simulink model "model_v4"  (R2023b)
settings: Solver=VariableStepAuto  StartTime=0.0  StopTime=10.0  RelTol=1e-3
(part 2 of 2)

== matlab function model_v4/MATLAB Function2 ==
  data: M input; y_m2_ddot output; m1 input; m2 input; m3 input; theta_m2 input; theta_m3 input; theta_M input; y_m2 input; y_M input; theta_m2_dot input; theta_m3_dot input; y_m2_dot input; y_M_dot input; y_M_ddot input; l1 input; l2 input; l3 input; r input; k1 input; k2 input; k3 input; k4 input; k5 input; c4 input; c5 input; Q3 input
function y_m2_ddot = y_m2(M, m1, m2, m3, theta_m2, theta_m3, theta_M, y_m2, y_M, theta_m2_dot, theta_m3_dot, y_m2_dot, y_M_dot, y_M_ddot, l1, l2, l3, r, k1, k2, k3, k4, k5, c4, c5, Q3)

g = 9.81;
y_m2_ddot = (M*g*sqrt((l3*sin(theta_m3) - y_M*tan(theta_M) + y_m2*tan(theta_M))^2 + (l1*theta_m2 + l3*cos(theta_m3) - y_M - y_m2)^2)*(l3*sin(theta_m3) - y_M*tan(theta_M) + y_m2*tan(theta_M))^2*cos(theta_M)*tan(theta_M) - M*g*sqrt((l3*sin(theta_m3) - y_M*tan(theta_M) + y_m2*tan(theta_M))^2 + (l1*theta_m2 + l3*cos(theta_m3) - y_M - y_m2)^2)*(l3*sin(theta_m3) - y_M*tan(theta_M) + y_m2*tan(theta_M))^2*tan(theta_M)^2 + M*g*sqrt((l3*sin(theta_m3) - y_M*tan(theta_M) + y_m2*tan(theta_M))^2 + (l1*theta_m2 + l3*cos(theta_m3) - y_M - y_m2)^2)*(l1*theta_m2 + l3*cos(theta_m3) - y_M - y_m2)^2*cos(theta_M)*tan(theta_M) - M*g*sqrt((l3*sin(theta_m3) - y_M*tan(theta_M) + y_m2*tan(theta_M))^2 + (l1*theta_m2 + l3*cos(theta_m3) - y_M - y_m2)^2)*(l1*theta_m2 + l3*cos(theta_m3) - y_M - y_m2)^2*tan(theta_M)^2 + Q3*sqrt((l3*sin(theta_m3) - y_M*tan(theta_M) + y_m2*tan(theta_M))^2 + (l1*theta_m2 + l3*cos(theta_m3) - y_M - y_m2)^2)*(l3*sin(theta_m3) - y_M*tan(theta_M) + y_m2*tan(theta_M))^2*tan(theta_M)^2 + Q3*sqrt((l3*sin(theta_m3) - y_M*tan(theta_M) + y_m2*tan(theta_M))^2 + (l1*theta_m2 + l3*cos(theta_m3) - y_M - y_m2)^2)*(l1*theta_m2 + l3*cos(theta_m3) - y_M - y_m2)^2*tan(theta_M)^2 + c4*l1^3*theta_m2^2*theta_m2_dot*sqrt((l3*sin(theta_m3) - y_M*tan(theta_M) + y_m2*tan(theta_M))^2 + (l1*theta_m2 + l3*cos(theta_m3) - y_M - y_m2)^2)*tan(theta_M)^2 - c4*l1^2*l3*theta_m2^2*theta_m3_dot*sqrt((l3*sin(theta_m3) - y_M*tan(theta_M) + y_m2*tan(theta_M))^2 + (l1*theta_m2 + l3*cos(theta_m3) - y_M - y_m2)^2)*sin(theta_m3)*tan(theta_M)^2 - c4*l1^2*l3*theta_m2*theta_m2_dot*sqrt((l3*sin(theta_m3) - y_M*tan(theta_M) + y_m2*tan(theta_M))^2 + (l1*theta_m2 + l3*cos(theta_m3) - y_M - y_m2)^2)*sin(theta_m3)*tan(theta_M)^3 + 2.0*c4*l1^2*l3*theta_m2*theta_m2_dot*sqrt((l3*sin(theta_m3) - y_M*tan(theta_M) + y_m2*tan(theta_M))^2 + (l1*theta_m2 + l3*cos(theta_m3) - y_M - y_m2)^2)*cos(theta_m3)*tan(theta_M)^2 - c4*l1^2*theta_m2^2*y_M_dot*sqrt((l3*sin(theta_m3) - y_M*tan(theta_M) + y_m2*tan(theta_M))^2 + (l1*theta_m2 + l3*cos(theta_m3) - y_M - y_m2)^2)*tan(theta_M)^2 - c4*l1^2*theta_m2^2*y_m2_dot*sqrt((l3*sin(theta_m3) - y_M*tan(theta_M) + y_m2*tan(theta_M))^2 + (l1*theta_m2 + l3*cos(theta_m3) - y_M - y_m2)^2)*tan(theta_M)^2 + c4*l1^2*theta_m2*theta_m2_dot*y_M*sqrt((l3*sin(theta_m3) - y_M*tan(theta_M) + y_m2*tan(theta_M))^2 + (l1*theta_m2 + l3*cos(theta_m3) - y_M - y_m2)^2)*tan(theta_M)^4 - 2.0*c4*l1^2*theta_m2*theta_m2_dot*y_M*sqrt((l3*sin(theta_m3) - y_M*tan(theta_M) + y_m2*tan(theta_M))^2 + (l1*theta_m2 + l3*cos(theta_m3) - y_M - y_m2)^2)*tan(theta_M)^2 - c4*l1^2*theta_m2*theta_m2_dot*y_m2*sqrt((l3*sin(theta_m3) - y_M*tan(theta_M) + y_m2*tan(theta_M))^2 + (l1*theta_m2 + l3*cos(theta_m3) - y_M - y_m2)^2)*tan(theta_M)^4 - 2.0*c4*l1^2*theta_m2*theta_m2_dot*y_m2*sqrt((l3*sin(theta_m3) - y_M*tan(theta_M) + y_m2*tan(theta_M))^2 + (l1*theta_m2 + l3*cos(theta_m3) - y_M - y_m2)^2)*tan(theta_M)^2 + c4*l1*l3^2*theta_m2*theta_m3_dot*sqrt((l3*sin(theta_m3) - y_M*tan(theta_M) + y_m2*tan(theta_M))^2 + (l1*theta_m2 + l3*cos(theta_m3) - y_M - y_m2)^2)*sin(theta_m3)^2*tan(theta_M)^3 - c4*l1*l3^2*theta_m2*theta_m3_dot*sqrt((l3*sin(theta_m3) - y_M*tan(theta_M) + y_m2*tan(theta_M))^2 + (l1*theta_m2 + l3*cos(theta_m3) - y_M - y_m2)^2)*sin(theta_m3)*cos(theta_m3)*tan(theta_M)^2 - c4*l1*l3^2*theta_m2_dot*sqrt((l3*sin(theta_m3) - y_M*tan(theta_M) + y_m2*tan(theta_M))^2 + (l1*theta_m2 + l3*cos(theta_m3) - y_M - y_m2)^2)*sin(theta_m3)*cos(theta_m3)*tan(theta_M)^3 + c4*l1*l3^2*theta_m2_dot*sqrt((l3*sin(theta_m3) - y_M*tan(theta_M) + y_m2*tan(theta_M))^2 + (l1*theta_m2 + l3*cos(theta_m3) - y_M - y_m2)^2)*cos(theta_m3)^2*tan(theta_M)^2 - c4*l1*l3*theta_m2*theta_m3_dot*y_M*sqrt((l3*sin(theta_m3) - y_M*tan(theta_M) + y_m2*tan(theta_M))^2 + (l1*theta_m2 + l3*cos(theta_m3) - y_M - y_m2)^2)*sin(theta_m3)*tan(theta_M)^4 + 2.0*c4*l1*l3*theta_m2*theta_m3_dot*y_M*sqrt((l3*sin(theta_m3) - y_M*tan(theta_M) + y_m2*tan(theta_M))^2 + (l1*theta_m2 + l3*cos(theta_m3) - y_M - y_m2)^2)*sin(theta_m3)*tan(theta_M)^2 - c4*l1*l3*theta_m2*theta_m3_dot*y_M*sqrt((l3*sin(theta_m3) - y_M*tan(theta_M) + y_m2*tan(theta_M))^2 + (l1*theta_m2 + l3*cos(theta_m3) - y_M - y_m2)^2)*cos(theta_m3)*tan(theta_M)^3 + c4*l1*l3*theta_m2*theta_m3_dot*y_m2*sqrt((l3*sin(theta_m3) - y_M*tan(theta_M) + y_m2*tan(theta_M))^2 + (l1*theta_m2 + l3*cos(theta_m3) - y_M - y_m2)^2)*sin(theta_m3)*tan(theta_M)^4 + 2.0*c4*l1*l3*theta_m2*theta_m3_dot*y_m2*sqrt((l3*sin(theta_m3) - y_M*tan(theta_M) + y_m2*tan(theta_M))^2 + (l1*theta_m2 + l3*cos(theta_m3) - y_M - y_m2)^2)*sin(theta_m3)*tan(theta_M)^2 + c4*l1*l3*theta_m2*theta_m3_dot*y_m2*sqrt((l3*sin(theta_m3) - y_M*tan(theta_M) + y_m2*tan(theta_M))^2 + (l1*theta_m2 + l3*cos(theta_m3) - y_M - y_m2)^2)*cos(theta_m3)*tan(theta_M)^3 - 2.0*c4*l1*l3*theta_m2*y_M_dot*sqrt((l3*sin(theta_m3) - y_M*tan(theta_M) + y_m2*tan(theta_M))^2 + (l1*theta_m2 + l3*cos(theta_m3) - y_M - y_m2)^2)*cos(theta_m3)*tan(theta_M)^2 + 2.0*c4*l1*l3*theta_m2*y_m2_dot*sqrt((l3*sin(theta_m3) - y_M*tan(theta_M) + y_m2*tan(theta_M))^2 + (l1*theta_m2 + l3*cos(theta_m3) - y_M - y_m2)^2)*sin(theta_m3)*tan(theta_M)^3 - 2.0*c4*l1*l3*theta_m2*y_m2_dot*sqrt((l3*sin(theta_m3) - y_M*tan(theta_M) + y_m2*tan(theta_M))^2 + (l1*theta_m2 + l3*cos(theta_m3) - y_M - y_m2)^2)*cos(theta_m3)*tan(theta_M)^2 + c4*l1*l3*theta_m2_dot*y_M*sqrt((l3*sin(theta_m3) - y_M*tan(theta_M) + y_m2*tan(theta_M))^2 + (l1*theta_m2 + l3*cos(theta_m3) - y_M - y_m2)^2)*sin(theta_m3)*tan(theta_M)^3 + c4*l1*l3*theta_m2_dot*y_M*sqrt((l3*sin(theta_m3) - y_M*tan(theta_M) + y_m2*tan(theta_M))^2 + (l1*theta_m2 + l3*cos(theta_m3) - y_M - y_m2)^2)*cos(theta_m3)*tan(theta_M)^4 - 2.0*c4*l1*l3*theta_m2_dot*y_M*sqrt((l3*sin(theta_m3) - y_M*tan(theta_M) + y_m2*tan(theta_M))^2 + (l1*theta_m2 + l3*cos(theta_m3) - y_M - y_m2)^2)*cos(theta_m3)*tan(theta_M)^2 + c4*l1*l3*theta_m2_dot*y_m2*sqrt((l3*sin(theta_m3) - y_M*tan(theta_M) + y_m2*tan(theta_M))^2 + (l1*theta_m2 + l3*cos(theta_m3) - y_M - y_m2)^2)*sin(theta_m3)*tan(theta_M)^3 - c4*l1*l3*theta_m2_dot*y_m2*sqrt((l3*sin(theta_m3) - y_M*tan(theta_M) + y_m2*tan(theta_M))^2 + (l1*theta_m2 + l3*cos(theta_m3) - y_M - y_m2)^2)*cos(theta_m3)*tan(theta_M)^4 - 2.0*c4*l1*l3*theta_m2_dot*y_m2*sqrt((l3*sin(theta_m3) - y_M*tan(theta_M) + y_m2*tan(theta_M))^2 + (l1*theta_m2 + l3*cos(theta_m3) - y_M - y_m2)^2)*cos(theta_m3)*tan(theta_M)^2 + 2.0*c4*l1*theta_m2*y_M*y_M_dot*sqrt((l3*sin(theta_m3) - y_M*tan(theta_M) + y_m2*tan(theta_M))^2 + (l1*theta_m2 + l3*cos(theta_m3) - y_M - y_m2)^2)*tan(theta_M)^2 - 2.0*c4*l1*theta_m2*y_M*y_m2_dot*sqrt((l3*sin(theta_m3) - y_M*tan(theta_M) + y_m2*tan(theta_M))^2 + (l1*theta_m2 + l3*cos(theta_m3) - y_M - y_m2)^2)*tan(theta_M)^4 + 2.0*c4*l1*theta_m2*y_M*y_m2_dot*sqrt((l3*sin(theta_m3) - y_M*tan(theta_M) + y_m2*tan(theta_M))^2 + (l1*theta_m2 + l3*cos(theta_m3) - y_M - y_m2)^2)*tan(theta_M)^2 + 2.0*c4*l1*theta_m2*y_M_dot*y_m2*sqrt((l3*sin(theta_m3) - y_M*tan(theta_M) + y_m2*tan(theta_M))^2 + (l1*theta_m2 + l3*cos(theta_m3) - y_M - y_m2)^2)*tan(theta_M)^2 + 2.0*c4*l1*theta_m2*y_m2*y_m2_dot*sqrt((l3*sin(theta_m3) - y_M*tan(theta_M) + y_m2*tan(theta_M))^2 + (l1*theta_m2 + l3*cos(theta_m3) - y_M - y_m2)^2)*tan(theta_M)^4 + 2.0*c4*l1*theta_m2*y_m2*y_m2_dot*sqrt((l3*sin(theta_m3) - y_M*tan(theta_M) + y_m2*tan(theta_M))^2 + (l1*theta_m2 + l3*cos(theta_m3) - y_M - y_m2)^2)*tan(theta_M)^2 - c4*l1*theta_m2_dot*y_M^2*sqrt((l3*sin(theta_m3) - y_M*tan(theta_M) + y_m2*tan(theta_M))^2 + (l1*theta_m2 + l3*cos(theta_m3) - y_M - y_m2)^2)*tan(theta_M)^4 + c4*l1*theta_m2_dot*y_M^2*sqrt((l3*sin(theta_m3) - y_M*tan(theta_M) + y_m2*tan(theta_M))^2 + (l1*theta_m2 + l3*cos(theta_m3) - y_M - y_m2)^2)*tan(theta_M)^2 + 2.0*c4*l1*theta_m2_dot*y_M*y_m2*sqrt((l3*sin(theta_m3) - y_M*tan(theta_M) + y_m2*tan(theta_M))^2 + (l1*theta_m2 + l3*cos(theta_m3) - y_M - y_m2)^2)*tan(theta_M)^2 + c4*l1*theta_m2_dot*y_m2^2*sqrt((l3*sin(theta_m3) - y_M*tan(theta_M) + y_m2*tan(theta_M))^2 + (l1*theta_m2 + l3*cos(theta_m3) - y_M - y_m2)^2)*tan(theta_M)^4 + c4*l1*theta_m2_dot*y_m2^2*sqrt((l3*sin(theta_m3) - y_M*tan(theta_M) + y_m2*tan(theta_M))^2 + (l1*theta_m2 + l3*cos(theta_m3) - y_M - y_m2)^2)*tan(theta_M)^2 - c4*l3^2*theta_m3_dot*y_M*sqrt((l3*sin(theta_m3) - y_M*tan(theta_M) + y_m2*tan(theta_M))^2 + (l1*theta_m2 + l3*cos(theta_m3) - y_M - y_m2)^2)*sin(theta_m3)^2*tan(theta_M)^3 + c4*l3^2*theta_m3_dot*y_M*sqrt((l3*sin(theta_m3) - y_M*tan(theta_M) + y_m2*tan(theta_M))^2 + (l1*theta_m2 + l3*cos(theta_m3) - y_M - y_m2)^2)*sin(theta_m3)*cos(theta_m3)*tan(theta_M)^4 + c4*l3^2*theta_m3_dot*y_M*sqrt((l3*sin(theta_m3) - y_M*tan(theta_M) + y_m2*tan(theta_M))^2 + (l1*theta_m2 + l3*cos(theta_m3) - y_M - y_m2)^2)*sin(theta_m3)*cos(theta_m3)*tan(theta_M)^2 - c4*l3^2*theta_m3_dot*y_M*sqrt((l3*sin(theta_m3) - y_M*tan(theta_M) + y_m2*tan(theta_M))^2 + (l1*theta_m2 + l3*cos(theta_m3) - y_M - y_m2)^2)*cos(theta_m3)^2*tan(theta_M)^3 - c4*l3^2*theta_m3_dot*y_m2*sqrt((l3*sin(theta_m3) - y_M*tan(theta_M) + y_m2*tan(theta_M))^2 + (l1*theta_m2 + l3*cos(theta_m3) - y_M - y_m2)^2)*sin(theta_m3)^2*tan(theta_M)^3 - c4*l3^2*theta_m3_dot*y_m2*sqrt((l3*sin(theta_m3) - y_M*tan(theta_M) + y_m2*tan(theta_M))^2 + (l1*theta_m2 + l3*cos(theta_m3) - y_M - y_m2)^2)*sin(theta_m3)*cos(theta_m3)*tan(theta_M)^4 + c4*l3^2*theta_m3_dot*y_m2*sqrt((l3*sin(theta_m3) - y_M*tan(theta_M) + y_m2*tan(theta_M))^2 + (l1*theta_m2 + l3*cos(theta_m3) - y_M - y_m2)^2)*sin(theta_m3)*cos(theta_m3)*tan(theta_M)^2 + c4*l3^2*theta_m3_dot*y_m2*sqrt((l3*sin(theta_m3) - y_M*tan(theta_M) + y_m2*tan(theta_M))^2 + (l1*theta_m2 + l3*cos(theta_m3) - y_M - y_m2)^2)*cos(theta_m3)^2*tan(theta_M)^3 + c4*l3^2*y_M_dot*sqrt((l3*sin(theta_m3) - y_M*tan(theta_M) + y_m2*tan(theta_M))^2 + (l1*theta_m2 + l3*cos(theta_m3) - y_M - y_m2)^2)*sin(theta_m3)^2*tan(theta_M)^4 - c4*l3^2*y_M_dot*sqrt((l3*sin(theta_m3) - y_M*tan(theta_M) + y_m2*tan(theta_M))^2 + (l1*theta_m2 + l3*cos(theta_m3) - y_M - y_m2)^2)*cos(theta_m3)^2*tan(theta_M)^2 - c4*l3^2*y_m2_dot*sqrt((l3*sin(theta_m3) - y_M*tan(theta_M) + y_m2*tan(theta_M))^2 + (l1*theta_m2 + l3*cos(theta_m3) - y_M - y_m2)^2)*sin(theta_m3)^2*tan(theta_M)^4 + 2.0*c4*l3^2*y_m2_dot*sqrt((l3*sin(theta_m3) - y_M*tan(theta_M) + y_m2*tan(theta_M))^2 + (l1*theta_m2 + l3*cos(theta_m3) - y_M - y_m2)^2)*sin(theta_m3)*cos(theta_m3)*tan(theta_M)^3 - c4*l3^2*y_m2_dot*sqrt((l3*sin(theta_m3) - y_M*tan(theta_M) + y_m2*tan(theta_M))^2 + (l1*theta_m2 + l3*cos(theta_m3) - y_M - y_m2)^2)*cos(theta_m3)^2*tan(theta_M)^2 + c4*l3*theta_m3_dot*y_M^2*sqrt((l3*sin(theta_m3) - y_M*tan(theta_M) + y_m2*tan(theta_M))^2 + (l1*theta_m2 + l3*cos(theta_m3) - y_M - y_m2)^2)*sin(theta_m3)*tan(theta_M)^4 - c4*l3*theta_m3_dot*y_M^2*sqrt((l3*sin(theta_m3) - y_M*tan(theta_M) + y_m2*tan(theta_M))^2 + (l1*theta_m2 + l3*cos(theta_m3) - y_M - y_m2)^2)*sin(theta_m3)*tan(theta_M)^2 - c4*l3*theta_m3_dot*y_M^2*sqrt((l3*sin(theta_m3) - y_M*tan(theta_M) + y_m2*tan(theta_M))^2 + (l1*theta_m2 + l3*cos(theta_m3) - y_M - y_m2)^2)*cos(theta_m3)*tan(theta_M)^5 + c4*l3*theta_m3_dot*y_M^2*sqrt((l3*sin(theta_m3) - y_M*tan(theta_M) + y_m2*tan(theta_M))^2 + (l1*theta_m2 + l3*cos(theta_m3) - y_M - y_m2)^2)*cos(theta_m3)*tan(theta_M)^3 - 2.0*c4*l3*theta_m3_dot*y_M*y_m2*sqrt((l3*sin(theta_m3) - y_M*tan(theta_M) + y_m2*tan(theta_M))^2 + (l1*theta_m2 + l3*cos(theta_m3) - y_M - y_m2)^2)*sin(theta_m3)*tan(theta_M)^2 + 2.0*c4*l3*theta_m3_dot*y_M*y_m2*sqrt((l3*sin(theta_m3) - y_M*tan(theta_M) + y_m2*tan(theta_M))^2 + (l1*theta_m2 + l3*cos(theta_m3) - y_M - y_m2)^2)*cos(theta_m3)*tan(theta_M)^5 - c4*l3*theta_m3_dot*y_m2^2*sqrt((l3*sin(theta_m3) - y_M*tan(theta_M) + y_m2*tan(theta_M))^2 + (l1*theta_m2 + l3*cos(theta_m3) - y_M - y_m2)^2)*sin(theta_m3)*tan(theta_M)^4 - c4*l3*theta_m3_dot*y_m2^2*sqrt((l3*sin(theta_m3) - y_M*tan(theta_M) + y_m2*tan(theta_M))^2 + (l1*theta_m2 + l3*cos(theta_m3) - y_M - y_m2)^2)*sin(theta_m3)*tan(theta_M)^2 - c4*l3*theta_m3_dot*y_m2^2*sqrt((l3*sin(theta_m3) - y_M*tan(theta_M) + y_m2*tan(theta_M))^2 + (l1*theta_m2 + l3*cos(theta_m3) - y_M - y_m2)^2)*cos(theta_m3)*tan(theta_M)^5 - c4*l3*theta_m3_dot*y_m2^2*sqrt((l3*sin(theta_m3) - y_M*tan(theta_M) + y_m2*tan(theta_M))^2 + (l1*theta_m2 + l3*cos(theta_m3) - y_M - y_m2)^2)*cos(theta_m3)*tan(theta_M)^3 - 2.0*c4*l3*y_M*y_M_dot*sqrt((l3*sin(theta_m3) - y_M*tan(theta_M) + y_m2*tan(theta_M))^2 + (l1*theta_m2 + l3*cos(theta_m3) - y_M - y_m2)^2)*sin(theta_m3)*tan(theta_M)^5 + 2.0*c4*l3*y_M*y_M_dot*sqrt((l3*sin(theta_m3) - y_M*tan(theta_M) + y_m2*tan(theta_M))^2 + (l1*theta_m2 + l3*cos(theta_m3) - y_M - y_m2)^2)*cos(theta_m3)*tan(theta_M)^2 + 2.0*c4*l3*y_M*y_m2_dot*sqrt((l3*sin(theta_m3) - y_M*tan(theta_M) + y_m2*tan(theta_M))^2 + (l1*theta_m2 + l3*cos(theta_m3) - y_M - y_m2)^2)*sin(theta_m3)*tan(theta_M)^5 - 2.0*c4*l3*y_M*y_m2_dot*sqrt((l3*sin(theta_m3) - y_M*tan(theta_M) + y_m2*tan(theta_M))^2 + (l1*theta_m2 + l3*cos(theta_m3) - y_M - y_m2)^2)*sin(theta_m3)*tan(theta_M)^3 - 2.0*c4*l3*y_M*y_m2_dot*sqrt((l3*sin(theta_m3) - y_M*tan(theta_M) + y_m2*tan(theta_M))^2 + (l1*theta_m2 + l3*cos(theta_m3) - y_M - y_m2)^2)*cos(theta_m3)*tan(theta_M)^4 + 2.0*c4*l3*y_M*y_m2_dot*sqrt((l3*sin(theta_m3) - y_M*tan(theta_M) + y_m2*tan(theta_M))^2 + (l1*theta_m2 + l3*cos(theta_m3) - y_M - y_m2)^2)*cos(theta_m3)*tan(theta_M)^2 + 2.0*c4*l3*y_M_dot*y_m2*sqrt((l3*sin(theta_m3) - y_M*tan(theta_M) + y_m2*tan(theta_M))^2 + (l1*theta_m2 + l3*cos(theta_m3) - y_M - y_m2)^2)*sin(theta_m3)*tan(theta_M)^5 + 2.0*c4*l3*y_M_dot*y_m2*sqrt((l3*sin(theta_m3) - y_M*tan(theta_M) + y_m2*tan(theta_M))^2 + (l1*theta_m2 + l3*cos(theta_m3) - y_M - y_m2)^2)*cos(theta_m3)*tan(theta_M)^2 - 2.0*c4*l3*y_m2*y_m2_dot*sqrt((l3*sin(theta_m3) - y_M*tan(theta_M) + y_m2*tan(theta_M))^2 + (l1*theta_m2 + l3*cos(theta_m3) - y_M - y_m2)^2)*sin(theta_m3)*tan(theta_M)^5 - 2.0*c4*l3*y_m2*y_m2_dot*sqrt((l3*sin(theta_m3) - y_M*tan(theta_M) + y_m2*tan(theta_M))^2 + (l1*theta_m2 + l3*cos(theta_m3) - y_M - y_m2)^2)*sin(theta_m3)*tan(theta_M)^3 + 2.0*c4*l3*y_m2*y_m2_dot*sqrt((l3*sin(theta_m3) - y_M*tan(theta_M) + y_m2*tan(theta_M))^2 + (l1*theta_m2 + l3*cos(theta_m3) - y_M - y_m2)^2)*cos(theta_m3)*tan(theta_M)^4 + 2.0*c4*l3*y_m2*y_m2_dot*sqrt((l3*sin(theta_m3) - y_M*tan(theta_M) + y_m2*tan(theta_M))^2 + (l1*theta_m2 + l3*cos(theta_m3) - y_M - y_m2)^2)*cos(theta_m3)*tan(theta_M)^2 + c4*y_M^2*y_M_dot*sqrt((l3*sin(theta_m3) - y_M*tan(theta_M) + y_m2*tan(theta_M))^2 + (l1*theta_m2 + l3*cos(theta_m3) - y_M - y_m2)^2)*tan(theta_M)^6 - c4*y_M^2*y_M_dot*sqrt((l3*sin(theta_m3) - y_M*tan(theta_M) + y_m2*tan(theta_M))^2 + (l1*theta_m2 + l3*cos(theta_m3) - y_M - y_m2)^2)*tan(theta_M)^2 - c4*y_M^2*y_m2_dot*sqrt((l3*sin(theta_m3) - y_M*tan(theta_M) + y_m2*tan(theta_M))^2 + (l1*theta_m2 + l3*cos(theta_m3) - y_M - y_m2)^2)*tan(theta_M)^6 + 2.0*c4*y_M^2*y_m2_dot*sqrt((l3*sin(theta_m3) - y_M*tan(theta_M) + y_m2*tan(theta_M))^2 + (l1*theta_m2 + l3*cos(theta_m3) - y_M - y_m2)^2)*tan(theta_M)^4 - c4*y_M^2*y_m2_dot*sqrt((l3*sin(theta_m3) - y_M*tan(theta_M) + y_m2*tan(theta_M))^2 + (l1*theta_m2 + l3*cos(theta_m3) - y_M - y_m2)^2)*tan(theta_M)^2 - 2.0*c4*y_M*y_M_dot*y_m2*sqrt((l3*sin(theta_m3) - y_M*tan(theta_M) + y_m2*tan(theta_M))^2 + (l1*theta_m2 + l3*cos(theta_m3) - y_M - y_m2)^2)*tan(theta_M)^6 - 2.0*c4*y_M*y_M_dot*y_m2*sqrt((l3*sin(theta_m3) - y_M*tan(theta_M) + y_m2*tan(theta_M))^2 + (l1*theta_m2 + l3*cos(theta_m3) - y_M - y_m2)^2)*tan(theta_M)^2 + 2.0*c4*y_M*y_m2*y_m2_dot*sqrt((l3*sin(theta_m3) - y_M*tan(theta_M) + y_m2*tan(theta_M))^2 + (l1*theta_m2 + l3*cos(theta_m3) - y_M - y_m2)^2)*tan(theta_M)^6 - 2.0*c4*y_M*y_m2*y_m2_dot*sqrt((l3*sin(theta_m3) - y_M*tan(theta_M) + y_m2*tan(theta_M))^2 + (l1*theta_m2 + l3*cos(theta_m3) - y_M - y_m2)^2)*tan(theta_M)^2 + c4*y_M_dot*y_m2^2*sqrt((l3*sin(theta_m3) - y_M*tan(theta_M) + y_m2*tan(theta_M))^2 + (l1*theta_m2 + l3*cos(theta_m3) - y_M - y_m2)^2)*tan(theta_M)^6 - c4*y_M_dot*y_m2^2*sqrt((l3*sin(theta_m3) - y_M*tan(theta_M) + y_m2*tan(theta_M))^2 + (l1*theta_m2 + l3*cos(theta_m3) - y_M - y_m2)^2)*tan(theta_M)^2 - c4*y_m2^2*y_m2_dot*sqrt((l3*sin(theta_m3) - y_M*tan(theta_M) + y_m2*tan(theta_M))^2 + (l1*theta_m2 + l3*cos(theta_m3) - y_M - y_m2)^2)*tan(theta_M)^6 - 2.0*c4*y_m2^2*y_m2_dot*sqrt((l3*sin(theta_m3) - y_M*tan(theta_M) + y_m2*tan(theta_M))^2 + (l1*theta_m2 + l3*cos(theta_m3) - y_M - y_m2)^2)*tan(theta_M)^4 - c4*y_m2^2*y_m2_dot*sqrt((l3*sin(theta_m3) - y_M*tan(theta_M) + y_m2*tan(theta_M))^2 + (l1*theta_m2 + l3*cos(theta_m3) - y_M - y_m2)^2)*tan(theta_M)^2 + c5*y_M_dot*sqrt((l3*sin(theta_m3) - y_M*tan(theta_M) + y_m2*tan(theta_M))^2 + (l1*theta_m2 + l3*cos(theta_m3) - y_M - y_m2)^2)*(l3*sin(theta_m3) - y_M*tan(theta_M) + y_m2*tan(theta_M))^2 + c5*y_M_dot*sqrt((l3*sin(theta_m3) - y_M*tan(theta_M) + y_m2*tan(theta_M))^2 + (l1*theta_m2 + l3*cos(theta_m3) - y_M - y_m2)^2)*(l1*theta_m2 + l3*cos(theta_m3) - y_M - y_m2)^2 - c5*y_m2_dot*sqrt((l3*sin(theta_m3) - y_M*tan(theta_M) + y_m2*tan(theta_M))^2 + (l1*theta_m2 + l3*cos(theta_m3) - y_M - y_m2)^2)*(l3*sin(theta_m3) - y_M*tan(theta_M) + y_m2*tan(theta_M))^2 - c5*y_m2_dot*sqrt((l3*sin(theta_m3) - y_M*tan(theta_M) + y_m2*tan(theta_M))^2 + (l1*theta_m2 + l3*cos(theta_m3) - y_M - y_m2)^2)*(l1*theta_m2 + l3*cos(theta_m3) - y_M - y_m2)^2 - g*m1*sqrt((l3*sin(theta_m3) - y_M*tan(theta_M) + y_m2*tan(theta_M))^2 + (l1*theta_m2 + l3*cos(theta_m3) - y_M - y_m2)^2)*(l3*sin(theta_m3) - y_M*tan(theta_M) + y_m2*tan(theta_M))^2*tan(theta_M)^2 - g*m1*sqrt((l3*sin(theta_m3) - y_M*tan(theta_M) + y_m2*tan(theta_M))^2 + (l1*theta_m2 + l3*cos(theta_m3) - y_M - y_m2)^2)*(l1*theta_m2 + l3*cos(theta_m3) - y_M - y_m2)^2*tan(theta_M)^2 - g*m2*sqrt((l3*sin(theta_m3) - y_M*tan(theta_M) + y_m2*tan(theta_M))^2 + (l1*theta_m2 + l3*cos(theta_m3) - y_M - y_m2)^2)*(l3*sin(theta_m3) - y_M*tan(theta_M) + y_m2*tan(theta_M))^2*tan(theta_M)^2 - g*m2*sqrt((l3*sin(theta_m3) - y_M*tan(theta_M) + y_m2*tan(theta_M))^2 + (l1*theta_m2 + l3*cos(theta_m3) - y_M - y_m2)^2)*(l1*theta_m2 + l3*cos(theta_m3) - y_M - y_m2)^2*tan(theta_M)^2 - g*m3*sqrt((l3*sin(theta_m3) - y_M*tan(theta_M) + y_m2*tan(theta_M))^2 + (l1*theta_m2 + l3*cos(theta_m3) - y_M - y_m2)^2)*(l3*sin(theta_m3) - y_M*tan(theta_M) + y_m2*tan(theta_M))^2*tan(theta_M)^2 - g*m3*sqrt((l3*sin(theta_m3) - y_M*tan(theta_M) + y_m2*tan(theta_M))^2 + (l1*theta_m2 + l3*cos(theta_m3) - y_M - y_m2)^2)*(l1*theta_m2 + l3*cos(theta_m3) - y_M - y_m2)^2*tan(theta_M)^2 - k1*l1*sqrt((l3*sin(theta_m3) - y_M*tan(theta_M) + y_m2*tan(theta_M))^2 + (l1*theta_m2 + l3*cos(theta_m3) - y_M - y_m2)^2)*(l3*sin(theta_m3) - y_M*tan(theta_M) + y_m2*tan(theta_M))^2*sin(theta_m2)*tan(theta_M)^2 - k1*l1*sqrt((l3*sin(theta_m3) - y_M*tan(theta_M) + y_m2*tan(theta_M))^2 + (l1*theta_m2 + l3*cos(theta_m3) - y_M - y_m2)^2)*(l1*theta_m2 + l3*cos(theta_m3) - y_M - y_m2)^2*sin(theta_m2)*tan(theta_M)^2 - k1*y_m2*sqrt((l3*sin(theta_m3) - y_M*tan(theta_M) + y_m2*tan(theta_M))^2 + (l1*theta_m2 + l3*cos(theta_m3) - y_M - y_m2)^2)*(l3*sin(theta_m3) - y_M*tan(theta_M) + y_m2*tan(theta_M))^2*tan(theta_M)^2 - k1*y_m2*sqrt((l3*sin(theta_m3) - y_M*tan(theta_M) + y_m2*tan(theta_M))^2 + (l1*theta_m2 + l3*cos(theta_m3) - y_M - y_m2)^2)*(l1*theta_m2 + l3*cos(theta_m3) - y_M - y_m2)^2*tan(theta_M)^2 - k2*y_m2*sqrt((l3*sin(theta_m3) - y_M*tan(theta_M) + y_m2*tan(theta_M))^2 + (l1*theta_m2 + l3*cos(theta_m3) - y_M - y_m2)^2)*(l3*sin(theta_m3) - y_M*tan(theta_M) + y_m2*tan(theta_M))^2*tan(theta_M)^2 - k2*y_m2*sqrt((l3*sin(theta_m3) - y_M*tan(theta_M) + y_m2*tan(theta_M))^2 + (l1*theta_m2 + l3*cos(theta_m3) - y_M - y_m2)^2)*(l1*theta_m2 + l3*cos(theta_m3) - y_M - y_m2)^2*tan(theta_M)^2 + k3*l1*sqrt((l3*sin(theta_m3) - y_M*tan(theta_M) + y_m2*tan(theta_M))^2 + (l1*theta_m2 + l3*cos(theta_m3) - y_M - y_m2)^2)*(l3*sin(theta_m3) - y_M*tan(theta_M) + y_m2*tan(theta_M))^2*sin(theta_m2)*tan(theta_M)^2 + k3*l1*sqrt((l3*sin(theta_m3) - y_M*tan(theta_M) + y_m2*tan(theta_M))^2 + (l1*theta_m2 + l3*cos(theta_m3) - y_M - y_m2)^2)*(l1*theta_m2 + l3*cos(theta_m3) - y_M - y_m2)^2*sin(theta_m2)*tan(theta_M)^2 - k3*y_m2*sqrt((l3*sin(theta_m3) - y_M*tan(theta_M) + y_m2*tan(theta_M))^2 + (l1*theta_m2 + l3*cos(theta_m3) - y_M - y_m2)^2)*(l3*sin(theta_m3) - y_M*tan(theta_M) + y_m2*tan(theta_M))^2*tan(theta_M)^2 - k3*y_m2*sqrt((l3*sin(theta_m3) - y_M*tan(theta_M) + y_m2*tan(theta_M))^2 + (l1*theta_m2 + l3*cos(theta_m3) - y_M - y_m2)^2)*(l1*theta_m2 + l3*cos(theta_m3) - y_M - y_m2)^2*tan(theta_M)^2 - k4*l1*l3*theta_m2*(l3*sin(theta_m3) - y_M*tan(theta_M) + y_m2*tan(theta_M))^2*tan(theta_M)^2 - k4*l1*l3*theta_m2*(l1*theta_m2 + l3*cos(theta_m3) - y_M - y_m2)^2*tan(theta_M)^2 + k4*l1*theta_m2*sqrt((l3*sin(theta_m3) - y_M*tan(theta_M) + y_m2*tan(theta_M))^2 + (l1*theta_m2 + l3*cos(theta_m3) - y_M - y_m2)^2)*(l3*sin(theta_m3) - y_M*tan(theta_M) + y_m2*tan(theta_M))^2*tan(theta_M)^2 + k4*l1*theta_m2*sqrt((l3*sin(theta_m3) - y_M*tan(theta_M) + y_m2*tan(theta_M))^2 + (l1*theta_m2 + l3*cos(theta_m3) - y_M - y_m2)^2)*(l1*theta_m2 + l3*cos(theta_m3) - y_M - y_m2)^2*tan(theta_M)^2 + k4*l3^2*(l3*sin(theta_m3) - y_M*tan(theta_M) + y_m2*tan(theta_M))^2*sin(theta_m3)*tan(theta_M)^3 - k4*l3^2*(l3*sin(theta_m3) - y_M*tan(theta_M) + y_m2*tan(theta_M))^2*cos(theta_m3)*tan(theta_M)^2 + k4*l3^2*(l1*theta_m2 + l3*cos(theta_m3) - y_M - y_m2)^2*sin(theta_m3)*tan(theta_M)^3 - k4*l3^2*(l1*theta_m2 + l3*cos(theta_m3) - y_M - y_m2)^2*cos(theta_m3)*tan(theta_M)^2 - k4*l3*y_M*(l3*sin(theta_m3) - y_M*tan(theta_M) + y_m2*tan(theta_M))^2*tan(theta_M)^4 + k4*l3*y_M*(l3*sin(theta_m3) - y_M*tan(theta_M) + y_m2*tan(theta_M))^2*tan(theta_M)^2 - k4*l3*y_M*(l1*theta_m2 + l3*cos(theta_m3) - y_M - y_m2)^2*tan(theta_M)^4 + k4*l3*y_M*(l1*theta_m2 + l3*cos(theta_m3) - y_M - y_m2)^2*tan(theta_M)^2 + k4*l3*y_m2*(l3*sin(theta_m3) - y_M*tan(theta_M) + y_m2*tan(theta_M))^2*tan(theta_M)^4 + k4*l3*y_m2*(l3*sin(theta_m3) - y_M*tan(theta_M) + y_m2*tan(theta_M))^2*tan(theta_M)^2 + k4*l3*y_m2*(l1*theta_m2 + l3*cos(theta_m3) - y_M - y_m2)^2*tan(theta_M)^4 + k4*l3*y_m2*(l1*theta_m2 + l3*cos(theta_m3) - y_M - y_m2)^2*tan(theta_M)^2 - k4*l3*sqrt((l3*sin(theta_m3) - y_M*tan(theta_M) + y_m2*tan(theta_M))^2 + (l1*theta_m2 + l3*cos(theta_m3) - y_M - y_m2)^2)*(l3*sin(theta_m3) - y_M*tan(theta_M) + y_m2*tan(theta_M))^2*sin(theta_m3)*tan(theta_M)^3 + k4*l3*sqrt((l3*sin(theta_m3) - y_M*tan(theta_M) + y_m2*tan(theta_M))^2 + (l1*theta_m2 + l3*cos(theta_m3) - y_M - y_m2)^2)*(l3*sin(theta_m3) - y_M*tan(theta_M) + y_m2*tan(theta_M))^2*cos(theta_m3)*tan(theta_M)^2 - k4*l3*sqrt((l3*sin(theta_m3) - y_M*tan(theta_M) + y_m2*tan(theta_M))^2 + (l1*theta_m2 + l3*cos(theta_m3) - y_M - y_m2)^2)*(l1*theta_m2 + l3*cos(theta_m3) - y_M - y_m2)^2*sin(theta_m3)*tan(theta_M)^3 + k4*l3*sqrt((l3*sin(theta_m3) - y_M*tan(theta_M) + y_m2*tan(theta_M))^2 + (l1*theta_m2 + l3*cos(theta_m3) - y_M - y_m2)^2)*(l1*theta_m2 + l3*cos(theta_m3) - y_M - y_m2)^2*cos(theta_m3)*tan(theta_M)^2 + k4*y_M*sqrt((l3*sin(theta_m3) - y_M*tan(theta_M) + y_m2*tan(theta_M))^2 + (l1*theta_m2 + l3*cos(theta_m3) - y_M - y_m2)^2)*(l3*sin(theta_m3) - y_M*tan(theta_M) + y_m2*tan(theta_M))^2*tan(theta_M)^4 - k4*y_M*sqrt((l3*sin(theta_m3) - y_M*tan(theta_M) + y_m2*tan(theta_M))^2 + (l1*theta_m2 + l3*cos(theta_m3) - y_M - y_m2)^2)*(l3*sin(theta_m3) - y_M*tan(theta_M) + y_m2*tan(theta_M))^2*tan(theta_M)^2 + k4*y_M*sqrt((l3*sin(theta_m3) - y_M*tan(theta_M) + y_m2*tan(theta_M))^2 + (l1*theta_m2 + l3*cos(theta_m3) - y_M - y_m2)^2)*(l1*theta_m2 + l3*cos(theta_m3) - y_M - y_m2)^2*tan(theta_M)^4 - k4*y_M*sqrt((l3*sin(theta_m3) - y_M*tan(theta_M) + y_m2*tan(theta_M))^2 + (l1*theta_m2 + l3*cos(theta_m3) - y_M - y_m2)^2)*(l1*theta_m2 + l3*cos(theta_m3) - y_M - y_m2)^2*tan(theta_M)^2 - k4*y_m2*sqrt((l3*sin(theta_m3) - y_M*tan(theta_M) + y_m2*tan(theta_M))^2 + (l1*theta_m2 + l3*cos(theta_m3) - y_M - y_m2)^2)*(l3*sin(theta_m3) - y_M*tan(theta_M) + y_m2*tan(theta_M))^2*tan(theta_M)^4 - k4*y_m2*sqrt((l3*sin(theta_m3) - y_M*tan(theta_M) + y_m2*tan(theta_M))^2 + (l1*theta_m2 + l3*cos(theta_m3) - y_M - y_m2)^2)*(l3*sin(theta_m3) - y_M*tan(theta_M) + y_m2*tan(theta_M))^2*tan(theta_M)^2 - k4*y_m2*sqrt((l3*sin(theta_m3) - y_M*tan(theta_M) + y_m2*tan(theta_M))^2 + (l1*theta_m2 + l3*cos(theta_m3) - y_M - y_m2)^2)*(l1*theta_m2 + l3*cos(theta_m3) - y_M - y_m2)^2*tan(theta_M)^4 - k4*y_m2*sqrt((l3*sin(theta_m3) - y_M*tan(theta_M) + y_m2*tan(theta_M))^2 + (l1*theta_m2 + l3*cos(theta_m3) - y_M - y_m2)^2)*(l1*theta_m2 + l3*cos(theta_m3) - y_M - y_m2)^2*tan(theta_M)^2 + k5*y_M*sqrt((l3*sin(theta_m3) - y_M*tan(theta_M) + y_m2*tan(theta_M))^2 + (l1*theta_m2 + l3*cos(theta_m3) - y_M - y_m2)^2)*(l3*sin(theta_m3) - y_M*tan(theta_M) + y_m2*tan(theta_M))^2 + k5*y_M*sqrt((l3*sin(theta_m3) - y_M*tan(theta_M) + y_m2*tan(theta_M))^2 + (l1*theta_m2 + l3*cos(theta_m3) - y_M - y_m2)^2)*(l1*theta_m2 + l3*cos(theta_m3) - y_M - y_m2)^2 - k5*y_m2*sqrt((l3*sin(theta_m3) - y_M*tan(theta_M) + y_m2*tan(theta_M))^2 + (l1*theta_m2 + l3*cos(theta_m3) - y_M - y_m2)^2)*(l3*sin(theta_m3) - y_M*tan(theta_M) + y_m2*tan(theta_M))^2 - k5*y_m2*sqrt((l3*sin(theta_m3) - y_M*tan(theta_M) + y_m2*tan(theta_M))^2 + (l1*theta_m2 + l3*cos(theta_m3) - y_M - y_m2)^2)*(l1*theta_m2 + l3*cos(theta_m3) - y_M - y_m2)^2 + m1*y_M_ddot*sqrt((l3*sin(theta_m3) - y_M*tan(theta_M) + y_m2*tan(theta_M))^2 + (l1*theta_m2 + l3*cos(theta_m3) - y_M - y_m2)^2)*(l3*sin(theta_m3) - y_M*tan(theta_M) + y_m2*tan(theta_M))^2*tan(theta_M)^4 + m1*y_M_ddot*sqrt((l3*sin(theta_m3) - y_M*tan(theta_M) + y_m2*tan(theta_M))^2 + (l1*theta_m2 + l3*cos(theta_m3) - y_M - y_m2)^2)*(l1*theta_m2 + l3*cos(theta_m3) - y_M - y_m2)^2*tan(theta_M)^4 + m2*y_M_ddot*sqrt((l3*sin(theta_m3) - y_M*tan(theta_M) + y_m2*tan(theta_M))^2 + (l1*theta_m2 + l3*cos(theta_m3) - y_M - y_m2)^2)*(l3*sin(theta_m3) - y_M*tan(theta_M) + y_m2*tan(theta_M))^2*tan(theta_M)^4 + m2*y_M_ddot*sqrt((l3*sin(theta_m3) - y_M*tan(theta_M) + y_m2*tan(theta_M))^2 + (l1*theta_m2 + l3*cos(theta_m3) - y_M - y_m2)^2)*(l1*theta_m2 + l3*cos(theta_m3) - y_M - y_m2)^2*tan(theta_M)^4 + m3*y_M_ddot*sqrt((l3*sin(theta_m3) - y_M*tan(theta_M) + y_m2*tan(theta_M))^2 + (l1*theta_m2 + l3*cos(theta_m3) - y_M - y_m2)^2)*(l3*sin(theta_m3) - y_M*tan(theta_M) + y_m2*tan(theta_M))^2*tan(theta_M)^4 + m3*y_M_ddot*sqrt((l3*sin(theta_m3) - y_M*tan(theta_M) + y_m2*tan(theta_M))^2 + (l1*theta_m2 + l3*cos(theta_m3) - y_M - y_m2)^2)*(l1*theta_m2 + l3*cos(theta_m3) - y_M - y_m2)^2*tan(theta_M)^4)/(sqrt((l3*sin(theta_m3) - y_M*tan(theta_M) + y_m2*tan(theta_M))^2 + (l1*theta_m2 + l3*cos(theta_m3) - y_M - y_m2)^2)*(m1*(l3*sin(theta_m3) - y_M*tan(theta_M) + y_m2*tan(theta_M))^2*tan(theta_M)^2 + m1*(l1*theta_m2 + l3*cos(theta_m3) - y_M - y_m2)^2*tan(theta_M)^2 + m2*(l3*sin(theta_m3) - y_M*tan(theta_M) + y_m2*tan(theta_M))^2*tan(theta_M)^2 + m2*(l3*sin(theta_m3) - y_M*tan(theta_M) + y_m2*tan(theta_M))^2 + m2*(l1*theta_m2 + l3*cos(theta_m3) - y_M - y_m2)^2*tan(theta_M)^2 + m2*(l1*theta_m2 + l3*cos(theta_m3) - y_M - y_m2)^2 + m3*(l3*sin(theta_m3) - y_M*tan(theta_M) + y_m2*tan(theta_M))^2*tan(theta_M)^2 + m3*(l1*theta_m2 + l3*cos(theta_m3) - y_M - y_m2)^2*tan(theta_M)^2)*tan(theta_M)^2);
